simulink model "transfert_function"  (R2024b)
settings: Solver=ode1  StartTime=0.0  StopTime=inf  FixedStep=dt  MaxStep=1/30  RelTol=1e-3
undefined symbols (not defined in the file or in its folder): f, Kb, Kd, Ki, Kp, p0
libraries: instrumentlib x2, simulink x1
settings Model: Creator=aalessan  LastModifiedBy=aalessan

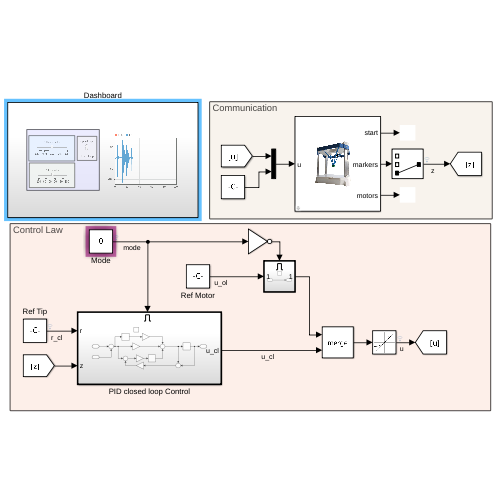
[thumbnail: Simulink's stored preview of the top-level diagram]
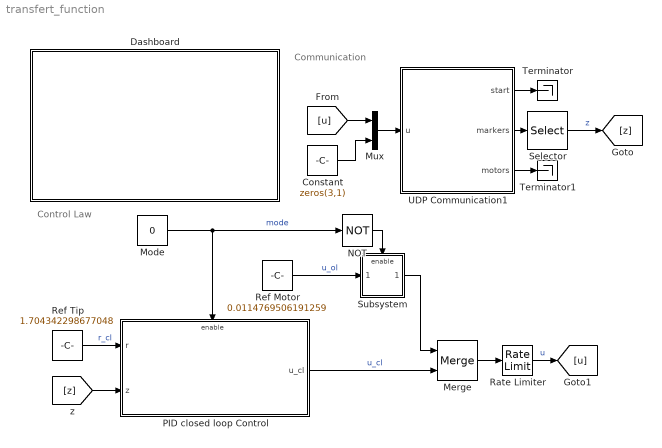
== system transfert_function ==
  note: Communication
  note: Control Law
  Constant : Constant  Value=zeros(3,1)
  Dashboard : Subsystem
  Merge : Merge  InitialOutput=zeros(1,1)
  Mode : Constant  Value=0
  Mux : Mux  Inputs=2
  NOT : Logic  Operator=NOT  IconShape=distinctive  AllPortsSameDT=off  OutDataTypeStr=boolean
  PID closed loop Control : Subsystem
  Rate Limiter : RateLimiter  RisingSlewLimit=7.906  FallingSlewLimit=-7.906  SampleTimeMode=inherited
  Ref Motor : Constant  Value=0.0114769506191259
  Ref Tip : Constant  Value=1.704342298677048
  Selector : Selector  InputPortWidth=3  IndexOptions=Index vector (dialog)  Indices=[3]  OutputSizes=1
  Subsystem : Subsystem
  Terminator : Terminator
  Terminator1 : Terminator
  UDP Communication1 : Subsystem  mask{nb_markers=1, markers_init=p0}
      mask prompts: nb_markers "Nb Markers"; markers_init "Initial Markers Position"
      mask Display: image('emio.png', [0,0,10,0,50,50]);
  wires:
  Ref Tip/1 -> PID closed loop Control/1(r)  "r_cl"
  NOT/1 -> Subsystem/Enable
  Rate Limiter/1 -> [u]  "u"
  Ref Motor/1 -> Subsystem/1(In1)  "u_ol"
  [z] -> PID closed loop Control/2(z)
  Mode/1 -> NOT/1, PID closed loop Control/Enable  "mode"
  Merge/1 -> Rate Limiter/1
  Subsystem/1(Out1) -> Merge/1
  PID closed loop Control/1(u_cl) -> Merge/2  "u_cl"
  [u] -> Mux/1
  Mux/1 -> UDP Communication1/1(u)
  Constant/1 -> Mux/2
  UDP Communication1/1(start) -> Terminator/1
  UDP Communication1/3(motors) -> Terminator1/1
  UDP Communication1/2(markers) -> Selector/1
  Selector/1 -> [z]  "z"

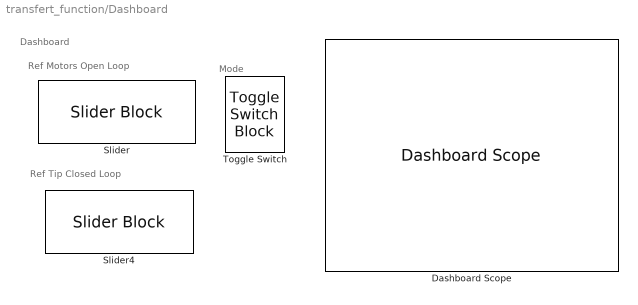
== system transfert_function/Dashboard ==
  note: Mode
  note: Ref Tip Closed Loop
  note: Dashboard
  note: Ref Motors Open Loop
  Dashboard Scope : DashboardScope  Ymin=-50  Ymax=50  UpdateMode=Scroll
  Slider : SliderBlock  ScaleMin=-1.57  ScaleMax=1.57
  Slider4 : SliderBlock  ScaleMin=-100
  Toggle Switch : ToggleSwitchBlock  LabelPosition=Hide
      settings: Values={{'Closed Loop', 'Open Loop'}, [1 0]}

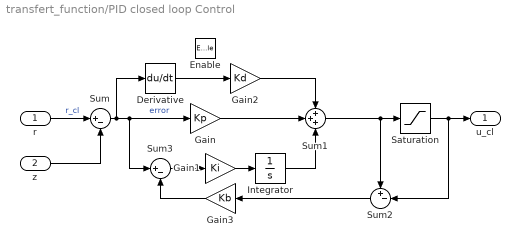
== system transfert_function/PID closed loop Control ==
  r : Inport
  z : Inport  Port=2
  Enable : EnablePort  StatesWhenEnabling=reset
  Derivative : Derivative
  Gain : Gain  Gain=Kp
  Gain1 : Gain  Gain=Ki
  Gain2 : Gain  Gain=Kd
  Gain3 : Gain  Gain=Kb
  Integrator : Integrator
  Saturation : Saturate  UpperLimit=1.57  LowerLimit=-1.57
  Sum : Sum  Inputs=|+-
  Sum1 : Sum  Inputs=+++
  Sum2 : Sum  Inputs=+-|
  Sum3 : Sum  Inputs=|+-
  u_cl : Outport
  wires:
  r/1 -> Sum/1  "r_cl"
  z/1 -> Sum/2
  Sum/1 -> Derivative/1, Gain/1, Sum3/1  "error"
  Saturation/1 -> Sum2/2, u_cl/1
  Sum3/1 -> Gain1/1
  Sum2/1 -> Gain3/1
  Sum1/1 -> Sum2/1, Saturation/1
  Gain2/1 -> Sum1/1
  Gain1/1 -> Integrator/1
  Gain3/1 -> Sum3/2
  Gain/1 -> Sum1/2
  Integrator/1 -> Sum1/3
  Derivative/1 -> Gain2/1

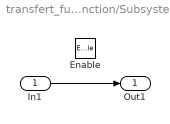
== system transfert_function/Subsystem ==
  In1 : Inport
  Enable : EnablePort
  Out1 : Outport
  wires:
  In1/1 -> Out1/1

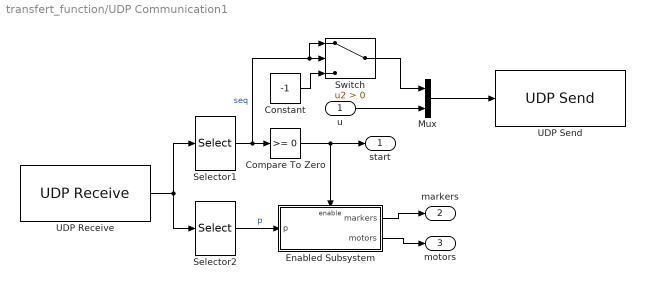
== system transfert_function/UDP Communication1 ==
  u : Inport
  Compare To Zero : simulink/Logic and Bit Operations/Compare To Zero  relop=>=  OutDataTypeStr=boolean
  Constant : Constant  Value=-1
  Enabled Subsystem : Subsystem  TreatAsAtomicUnit=on
  Mux : Mux  Inputs=2
  Selector1 : Selector  InputPortWidth=5+3*nb_markers  IndexOptions=Index vector (dialog)  Indices=[1]  OutputSizes=1
  Selector2 : Selector  InputPortWidth=5+3*nb_markers  IndexOptions=Index vector (dialog)  Indices=2:5+3*nb_markers  OutputSizes=1
  Switch : Switch  Criteria=u2 > Threshold  SaturateOnIntegerOverflow=off  InputSameDT=off
  UDP Receive : instrumentlib/UDP Receive  LocalAddress=127.0.0.1  LocalPort=25000  EnablePortSharing=off  Host=127.0.0.1  Port=9090  GetLatestData=on  DataSize=[ 3*nb_markers+5, 1 ]  DataType=double  ASCIIFormatting=%f,  Terminator=LF  CustomTerminator=10  ByteOrder=little-endian  EnableBlockingMode=on  Timeout=0.1  SampleTime=-1  SimulateUsing=Interpreted execution
  UDP Send : instrumentlib/UDP Send  Host=127.0.0.1  Port=25001  LocalAddress=0.0.0.0  LocalPort=-1  EnablePortSharing=off  OutputDatagramPacketSize=512  ByteOrder=little-endian  EnableBlockingMode=on  SimulateUsing=Interpreted execution
  start : Outport
  markers : Outport  Port=2
  motors : Outport  Port=3
  wires:
  Mux/1 -> UDP Send/1
  u/1 -> Mux/2
  Enabled Subsystem/2(motors) -> motors/1
  Selector2/1 -> Enabled Subsystem/1(p)  "p"
  Enabled Subsystem/1(markers) -> markers/1
  Selector1/1 -> Switch/1, Switch/2, Compare To Zero/1  "seq"
  Compare To Zero/1 -> start/1, Enabled Subsystem/Enable
  Constant/1 -> Switch/3
  UDP Receive/1 -> Selector1/1, Selector2/1
  Switch/1 -> Mux/1

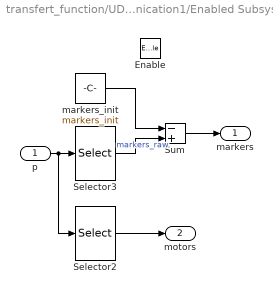
== system transfert_function/UDP Communication1/Enabled Subsystem ==
  p : Inport
  Enable : EnablePort
  Selector2 : Selector  InputPortWidth=4+3*nb_markers  IndexOptions=Index vector (dialog)  Indices=3*nb_markers+1:4+3*nb_markers  OutputSizes=1
  Selector3 : Selector  InputPortWidth=4+3*nb_markers  IndexOptions=Index vector (dialog)  Indices=1:3*nb_markers  OutputSizes=1
  Sum : Sum  Inputs=-+
  markers_init : Constant  Value=markers_init
  markers : Outport
  motors : Outport  Port=2
  wires:
  Sum/1 -> markers/1
  p/1 -> Selector2/1, Selector3/1
  Selector2/1 -> motors/1
  markers_init/1 -> Sum/1
  Selector3/1 -> Sum/2  "markers_raw"
